simulink model "sm_car_4post_testrig"  (R2021b)
settings: Solver=ode23t  StartTime=0.0  StopTime=20  MaxStep=0.4  RelTol=1e-3  AbsTol=1e-3  EnableMultiTasking=on
PreLoadFcn:
  | sm_car_4post_param
  | sm_car_4post_param_posts
  | load sm_car_4post_op_01
  | load sm_car_4post_op_02
  | load sm_car_4post_op_03
  | 
  | 
  | sm_car_4post_vehicle_01_data
  | sm_car_4post_vehicle_02_data
  | sm_car_4post_vehicle_03_data
  | sm_car_4post_init_data
  | Vehicle = Vehicle_01;
  | sm_car_4post_op = sm_car_4post_op_01;
values from neighbouring files (symbols this model uses):
  brake_pressure_factor = 0.1    [sm_car_4post_param.m]
  brake_rear_factor = 0.3    [sm_car_4post_param.m]
  Init = struct    [sm_car_4post_init_data.m]
  N = 100    [sm_extr_data_cam_roller_curve.m]
  s = sin(q)    [sm_extr_data_cam_roller_curve.m]
  sm_car_4post_op_01 = simscape.op.create(simlog_sm_car_4post,20)    [sm_car_4post_gen_op.m]
  Vehicle_01 = struct    [sm_car_4post_vehicle_01_data.m]
undefined symbols (not defined in the file or in its folder): Axle, Hub, ShaftF, ShaftR, smcar_param, X, xy_data_car_side, xy_data_membrane, Y, Z
libraries: fl_lib x68, sm_lib x50, nesl_utility x40, sm_car_4post_lib x34, simulink x2
(part 2 of 4)

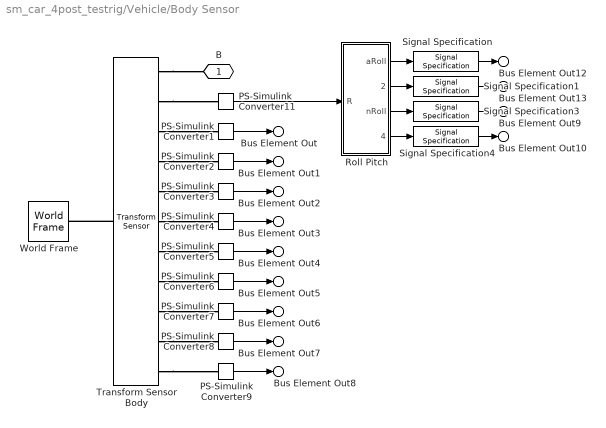
== system sm_car_4post_testrig/Vehicle/Body Sensor ==
  PS-Simulink Converter1 : nesl_utility/PS-Simulink Converter  PhysicalDomain=network_engine_domain  SubClassName=ps_output  LeftPortType=input  RightPortType=output  PseudoPeriodic=off  Frequencies=[]  Unit=m  AffineConversion=off
      settings: SourceProductBaseCode=PW,SS
  PS-Simulink Converter11 : nesl_utility/PS-Simulink Converter  PhysicalDomain=network_engine_domain  SubClassName=ps_output  LeftPortType=input  RightPortType=output  PseudoPeriodic=off  Frequencies=[]  Unit=1  AffineConversion=off
      settings: SourceProductBaseCode=PW,SS
  PS-Simulink Converter2 : nesl_utility/PS-Simulink Converter  PhysicalDomain=network_engine_domain  SubClassName=ps_output  LeftPortType=input  RightPortType=output  PseudoPeriodic=off  Frequencies=[]  Unit=m  AffineConversion=off
      settings: SourceProductBaseCode=PW,SS
  PS-Simulink Converter3 : nesl_utility/PS-Simulink Converter  PhysicalDomain=network_engine_domain  SubClassName=ps_output  LeftPortType=input  RightPortType=output  PseudoPeriodic=off  Frequencies=[]  Unit=m  AffineConversion=off
      settings: SourceProductBaseCode=PW,SS
  PS-Simulink Converter4 : nesl_utility/PS-Simulink Converter  PhysicalDomain=network_engine_domain  SubClassName=ps_output  LeftPortType=input  RightPortType=output  PseudoPeriodic=off  Frequencies=[]  Unit=m/s  AffineConversion=off
      settings: SourceProductBaseCode=PW,SS
  PS-Simulink Converter5 : nesl_utility/PS-Simulink Converter  PhysicalDomain=network_engine_domain  SubClassName=ps_output  LeftPortType=input  RightPortType=output  PseudoPeriodic=off  Frequencies=[]  Unit=m/s  AffineConversion=off
      settings: SourceProductBaseCode=PW,SS
  PS-Simulink Converter6 : nesl_utility/PS-Simulink Converter  PhysicalDomain=network_engine_domain  SubClassName=ps_output  LeftPortType=input  RightPortType=output  PseudoPeriodic=off  Frequencies=[]  Unit=m/s  AffineConversion=off
      settings: SourceProductBaseCode=PW,SS
  PS-Simulink Converter7 : nesl_utility/PS-Simulink Converter  PhysicalDomain=network_engine_domain  SubClassName=ps_output  LeftPortType=input  RightPortType=output  PseudoPeriodic=off  Frequencies=[]  Unit=m/s^2  AffineConversion=off
      settings: SourceProductBaseCode=PW,SS
  PS-Simulink Converter8 : nesl_utility/PS-Simulink Converter  PhysicalDomain=network_engine_domain  SubClassName=ps_output  LeftPortType=input  RightPortType=output  PseudoPeriodic=off  Frequencies=[]  Unit=m/s^2  AffineConversion=off
      settings: SourceProductBaseCode=PW,SS
  PS-Simulink Converter9 : nesl_utility/PS-Simulink Converter  PhysicalDomain=network_engine_domain  SubClassName=ps_output  LeftPortType=input  RightPortType=output  PseudoPeriodic=off  Frequencies=[]  Unit=m/s^2  AffineConversion=off
      settings: SourceProductBaseCode=PW,SS
  Roll Pitch : Subsystem
  Signal Specification : SignalSpecification  Unit=rad
  Signal Specification1 : SignalSpecification  Unit=rad
  Signal Specification3 : SignalSpecification  Unit=rad/s
  Signal Specification4 : SignalSpecification  Unit=rad/s
  Transform Sensor Body : sm_lib/Frames and Transforms/Transform Sensor  MeasurementFrame=NonRotatingFollower  SenseAngle=off  SenseAxis=off  SenseAngle1=off  SenseAngle2=off  SenseAngle3=off  SenseQ=off  SenseR=on  SenseOmegaX=off  SenseOmegaY=off  SenseOmegaZ=off  SenseOmega1=off  SenseOmega2=off  SenseOmega3=off  SenseQDot=off  SenseRDot=off  SenseAlphaX=off  SenseAlphaY=off  SenseAlphaZ=off  SenseAlpha1=off  SenseAlpha2=off  SenseAlpha3=off  SenseQDDot=off  SenseRDDot=off  SenseX=on  SenseY=on  SenseZ=on  SenseRad=off  SenseAzim=off  SenseDist=off  SenseInc=off  SenseXDot=on  SenseYDot=on  SenseZDot=on  SenseRadDot=off  SenseAzimDot=off  SenseDistDot=off  SenseIncDot=off  SenseXDDot=on  SenseYDDot=on  SenseZDDot=on  SenseRadDDot=off  SenseAzimDDot=off  SenseDistDDot=off  SenseIncDDot=off
  World Frame : sm_lib/Frames and Transforms/World Frame
  B : PMIOPort  Side=Left
  Bus Element Out : Outport  VectorParamsAs1DForOutWhenUnconnected=off  PortName=Body  Element=x
  Bus Element Out1 : Outport  VectorParamsAs1DForOutWhenUnconnected=off  PortName=Body  Element=y
  Bus Element Out2 : Outport  VectorParamsAs1DForOutWhenUnconnected=off  PortName=Body  Element=z
  Bus Element Out3 : Outport  VectorParamsAs1DForOutWhenUnconnected=off  PortName=Body  Element=vx
  Bus Element Out4 : Outport  VectorParamsAs1DForOutWhenUnconnected=off  PortName=Body  Element=vy
  Bus Element Out5 : Outport  VectorParamsAs1DForOutWhenUnconnected=off  PortName=Body  Element=vz
  Bus Element Out6 : Outport  VectorParamsAs1DForOutWhenUnconnected=off  PortName=Body  Element=gx
  Bus Element Out7 : Outport  VectorParamsAs1DForOutWhenUnconnected=off  PortName=Body  Element=gy
  Bus Element Out8 : Outport  VectorParamsAs1DForOutWhenUnconnected=off  PortName=Body  Element=gz
  Bus Element Out9 : Outport  VectorParamsAs1DForOutWhenUnconnected=off  PortName=Body  Element=nRoll
  Bus Element Out10 : Outport  VectorParamsAs1DForOutWhenUnconnected=off  PortName=Body  Element=nPitch
  Bus Element Out12 : Outport  VectorParamsAs1DForOutWhenUnconnected=off  PortName=Body  Element=aRoll
  Bus Element Out13 : Outport  VectorParamsAs1DForOutWhenUnconnected=off  PortName=Body  Element=aPitch
  wires:
  PS-Simulink Converter9/1 -> Bus Element Out8/1
  PS-Simulink Converter11/1 -> Roll Pitch/1(R)
  PS-Simulink Converter6/1 -> Bus Element Out5/1
  PS-Simulink Converter7/1 -> Bus Element Out6/1
  PS-Simulink Converter2/1 -> Bus Element Out1/1
  PS-Simulink Converter8/1 -> Bus Element Out7/1
  PS-Simulink Converter5/1 -> Bus Element Out4/1
  PS-Simulink Converter3/1 -> Bus Element Out2/1
  PS-Simulink Converter1/1 -> Bus Element Out/1
  PS-Simulink Converter4/1 -> Bus Element Out3/1
  Signal Specification/1 -> Bus Element Out12/1
  Signal Specification1/1 -> Bus Element Out13/1
  Signal Specification3/1 -> Bus Element Out9/1
  Signal Specification4/1 -> Bus Element Out10/1
  Roll Pitch/3(nRoll) -> Signal Specification3/1
  Roll Pitch/4(nPitch) -> Signal Specification4/1
  Roll Pitch/2(aPitch) -> Signal Specification1/1
  Roll Pitch/1(aRoll) -> Signal Specification/1
  connections:
  Transform Sensor Body/RConn5 -- PS-Simulink Converter3/LConn1
  Transform Sensor Body/RConn4 -- PS-Simulink Converter2/LConn1
  Transform Sensor Body/RConn11 -- PS-Simulink Converter9/LConn1
  Transform Sensor Body/RConn2 -- PS-Simulink Converter11/LConn1
  Transform Sensor Body/RConn7 -- PS-Simulink Converter5/LConn1
  Transform Sensor Body/RConn3 -- PS-Simulink Converter1/LConn1
  Transform Sensor Body/LConn1 -- World Frame/RConn1
  Transform Sensor Body/RConn1 -- B/RConn1
  Transform Sensor Body/RConn10 -- PS-Simulink Converter8/LConn1
  Transform Sensor Body/RConn9 -- PS-Simulink Converter7/LConn1
  Transform Sensor Body/RConn8 -- PS-Simulink Converter6/LConn1
  Transform Sensor Body/RConn6 -- PS-Simulink Converter4/LConn1

== system sm_car_4post_testrig/Vehicle/Brakes ==
  DrvBus : Inport
  CtrlBus : Inport  Port=2
  Pedal : Subsystem  Tag=PublishSubsystem  VariantControl=Pedal  mask(Pedal Controlled Brakes){brk_max_p_fa=Brakes.Front.Caliper.pMax.Value, brk_max_p_ra=Brakes.Rear.Caliper.pMax.Value, brk_filt_fa=1/Brakes.Front.Caliper.fActuatorCutoff.Value, brk_filt_ra=1/Brakes.Rear.Caliper.fActuatorCutoff.Value}
      mask help: Brakes for four-wheeled vehicle. The brake pressure varies with brake pedal travel (0-1).
      mask TypeOptions brk_max_p_fa: Actuator FL/brk_max_p | Actuator FR/brk_max_p
      mask TypeOptions brk_max_p_ra: Actuator RL/brk_max_p | Actuator RR/brk_max_p
      mask TypeOptions brk_filt_fa: Actuator FL/brk_filt | Actuator FR/brk_filt
      mask TypeOptions brk_filt_ra: Actuator RL/brk_filt | Actuator RR/brk_filt
      mask DialogControl cont_brakes Prompt: Brakes
      mask DialogControl cont_brk_act Prompt: Actuator
      mask DialogControl text_brakes_maxp Prompt: Max Pad Pressure (Pa)
      mask DialogControl text_brakes_filt Prompt: Time Constant (s)
  FL : PMIOPort  Side=Left
  FR : PMIOPort  Port=2  Side=Right
  RL : PMIOPort  Port=3  Side=Left
  RR : PMIOPort  Port=4  Side=Right
  BrakeOut : Outport  VectorParamsAs1DForOutWhenUnconnected=off
  wires:
  DrvBus/1 -> Pedal/1(DrvBus)
  Pedal/1(BrakeOut) -> BrakeOut/1
  CtrlBus/1 -> Pedal/2(CtrlBus)
  connections:
  Pedal/LConn1 -- FL/RConn1
  Pedal/RConn2 -- RR/RConn1
  Pedal/LConn2 -- RL/RConn1
  Pedal/RConn1 -- FR/RConn1

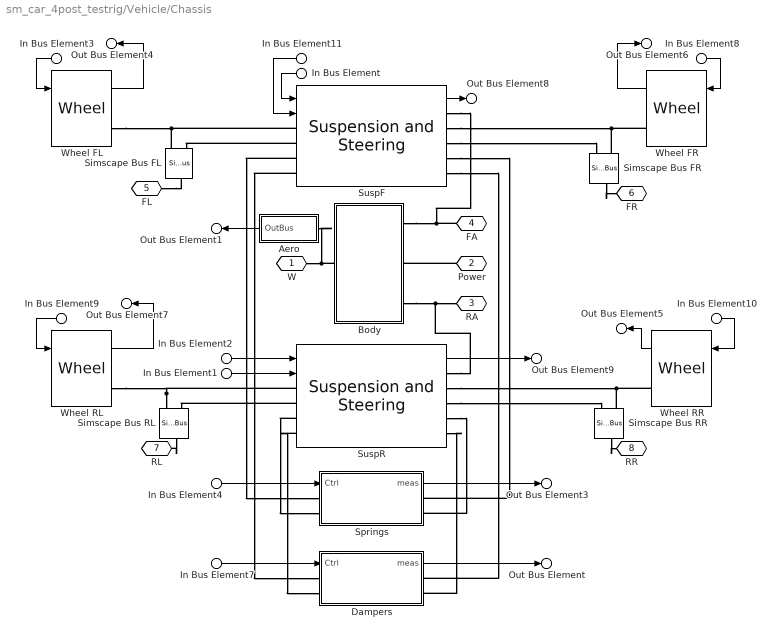
== system sm_car_4post_testrig/Vehicle/Chassis ==
  In Bus Element11 : Inport  PortName=DrvBus
  In Bus Element1 : Inport  PortName=DrvBus
  In Bus Element3 : Inport  Port=2  PortName=RdBus  Element=FL
  In Bus Element8 : Inport  Port=2  PortName=RdBus  Element=FR
  In Bus Element10 : Inport  Port=2  PortName=RdBus  Element=RR
  In Bus Element9 : Inport  Port=2  PortName=RdBus  Element=RL
  In Bus Element7 : Inport  Port=3  PortName=CtrlBus  Element=Damper
  In Bus Element : Inport  Port=3  PortName=CtrlBus  Element=SuspF
  In Bus Element2 : Inport  Port=3  PortName=CtrlBus  Element=SuspR
  In Bus Element4 : Inport  Port=3  PortName=CtrlBus  Element=Spring
  Aero : Subsystem  mask{CL=Chassis.Aero.CL.Value, CD=Chassis.Aero.CD.Value, rho=Chassis.Aero.rho_air.Value, A=Chassis.Aero.ARef.Value, sCentreOfPressure=Chassis.Aero.sPressureCentre.Value}
      mask prompts: CL "Lift Coeff (-)"; CD "Drag Coeff (-)"; rho "Air Density (kg/m^3)"; A "Reference Area (m^2)"; sCentreOfPressure "Centre of Pressure [xyz] (m)"
  Body : Subsystem  mask{hp_mount_fa=Chassis.Body.sAxleF.Value, hp_mount_ra=Chassis.Body.sAxleR.Value, hp_mount_power=Chassis.Body.sPower.Value, hp_chassis_cg=Chassis.Body.sCG.Value, chassis_mass=Chassis.Body.m.Value, chassis_inertia=Chassis.Body.J.Value, clr_chassis_hp_cg=smcar_param.hp.clr, opc_chassis_hp_cg=smcar_param.hp.opc, size_chassis_hp_cg=smcar_param.hp.rad, body_geo_hp=smcar_param.body.hp, whl_cutout_rad=0.5, whl_base=abs(Chassis.Body.sAxleF.Value(1)-Chassis.Body.sAxleR.Value(1)), thk_top=0.05, thk_side=0.05, car_track=Chassis.Body.Width.Value, extr_data_emblem_f=xy_data_membrane*0.2, extr_data_emblem_r=xy_data_membrane*0.2, clr_body_geo_top=smcar_param.blue, opc_body_geo_top=0.3*smcar_param.part.opc, clr_body_geo_left=smcar_param.blue, opc_body_geo_left=0.3*smcar_param.part.opc, clr_body_geo_right=smcar_param.blue, opc_body_geo_right=0.3*smcar_param.part.opc, clr_emblem_f=smcar_param.white, opc_emblem_f=smcar_param.part.opc, clr_emblem_r=smcar_param.white, opc_emblem_r=smcar_param.part.opc}
      mask prompts: hp_mount_power "HP Power [xyz] (m)"; hp_chassis_cg "Chassis CG [xyz] (m)"; chassis_mass "Mass (kg)"; chassis_inertia "Inertia [Ixx Iyy Izz]"; body_geo_hp "Body Geometry HP [xyz] (m)"; whl_cutout_rad "Wheel Cutout Radius (m)"; whl_base "Wheelbase (m)"; thk_top "Top Thickness (m)"; thk_side "Side Thickness (m)"; car_track "Width (m)"; extr_data_emblem_f "Emblem Data Front [xy] (m)"; extr_data_emblem_r "Emblem Data Rear [xy] (m)"
      mask TypeOptions hp_mount_fa:
      | Transform
      | Front Mount/TranslationCartesianOffset
      mask TypeOptions hp_mount_ra:
      | Transform
      | Rear Mount/TranslationCartesianOffset
      mask TypeOptions hp_mount_power:
      | Transform
      | Power Mount/TranslationCartesianOffset
      mask TypeOptions hp_chassis_cg:
      | Transform
      | Body CG/TranslationCartesianOffset
      mask TypeOptions chassis_mass:
      | Body Mass
      | and Inertia/Mass
      mask TypeOptions chassis_inertia:
      | Body Mass
      | and Inertia/MomentsOfInertia
      mask TypeOptions clr_chassis_hp_cg:
      | Body Mass
      | and Inertia/GraphicDiffuseColor | Vis HP Mount Front/GraphicDiffuseColor | Vis HP Mount Rear/GraphicDiffuseColor
      mask TypeOptions opc_chassis_hp_cg:
      | Body Mass
      | and Inertia/GraphicOpacity | Vis HP Mount Front/GraphicOpacity | Vis HP Mount Rear/GraphicOpacity
      mask TypeOptions size_chassis_hp_cg:
      | Body Mass
      | and Inertia/SphereRadius | Vis HP Mount Front/SphereRadius | Vis HP Mount Rear/SphereRadius
      mask TypeOptions body_geo_hp:
      | Transform
      | Body/TranslationCartesianOffset
      mask TypeOptions whl_cutout_rad:
      | Body
      | Geometry/whl_cutout_rad
      mask TypeOptions whl_base:
      | Body
      | Geometry/whl_base
      mask TypeOptions thk_top:
      | Body
      | Geometry/thk_top
      mask TypeOptions thk_side:
      | Body
      | Geometry/thk_side
      mask TypeOptions car_track:
      | Body
      | Geometry/car_track
      mask TypeOptions extr_data_emblem_f:
      | Body
      | Geometry/extr_data_emblem_f
      mask TypeOptions extr_data_emblem_r:
      | Body
      | Geometry/extr_data_emblem_r
      mask TypeOptions clr_body_geo_top:
      | Body
      | Geometry/clr_body_geo_top
      mask TypeOptions opc_body_geo_top:
      | Body
      | Geometry/opc_body_geo_top
      mask TypeOptions clr_body_geo_left:
      | Body
      | Geometry/clr_body_geo_left
      mask TypeOptions opc_body_geo_left:
      | Body
      | Geometry/opc_body_geo_left
      mask TypeOptions clr_body_geo_right:
      | Body
      | Geometry/clr_body_geo_right
      mask TypeOptions opc_body_geo_right:
      | Body
      | Geometry/opc_body_geo_right
      mask TypeOptions clr_emblem_f:
      | Body
      | Geometry/clr_emblem_f
      mask TypeOptions opc_emblem_f:
      | Body
      | Geometry/opc_emblem_f
      mask TypeOptions clr_emblem_r:
      | Body
      | Geometry/clr_emblem_r
      mask TypeOptions opc_emblem_r:
      | Body
      | Geometry/opc_emblem_r
      mask DialogControl cont_chassis Prompt: Chassis
      mask DialogControl text_chassis_mount_hp_blank Prompt: [xyz] (m)
      mask DialogControl text_chassis_fa Prompt: Front Susp.
      mask DialogControl text_chassis_ra Prompt: Rear Susp.
      mask DialogControl text_chassis_hp_mount Prompt: HP Mount
      mask DialogControl cont_chassis_vis Prompt: Visualization
      mask DialogControl text_chassis_vis_clr Prompt: Color [RGB]
      mask DialogControl text_chassis_vis_opc Prompt: Opacity (0-1)
      mask DialogControl text_chassis_vis_size Prompt: Size [xyz] (m)
      mask DialogControl text_chassis_vis_hp Prompt: Hardpoints
      mask DialogControl cont_body_geometry Prompt: Body
      mask DialogControl cont_body_geo_vis Prompt: Visualization
      mask DialogControl text_body_geo_clr Prompt: Color [RGB]
      mask DialogControl text_body_geo_opc Prompt: Opac. (0-1)
      mask DialogControl text_vis_body_geo_top Prompt: Top
      mask DialogControl text_vis_body_geo_l Prompt: Left Side
      mask DialogControl text_vis_body_geo_r Prompt: Right Side
      mask DialogControl text_vis_body_emblem_f Prompt: Emblem Front
      mask DialogControl text_vis_body_emblem_r Prompt: Emblem Rear
      mask Display: image(fullfile(matlabroot,'toolbox','physmod','sm','smdemos','car_4post_testrig','images','sm_car_4post_body_IMAGE.png'));
  Dampers : Subsystem  mask{Damper=Chassis.Damper}
      mask prompts: Damper "Damper Parameters"
      mask Display: image(fullfile(matlabroot,'toolbox','physmod','sm','smdemos','car_4post_testrig','images','sm_car_4post_damper_IMAGE.png'));
  Simscape Bus FL : SimscapeBus  HierarchyStrings=Axle;Hub
  Simscape Bus FR : SimscapeBus  HierarchyStrings=Hub;Axle
  Simscape Bus RL : SimscapeBus  HierarchyStrings=Axle;Hub
  Simscape Bus RR : SimscapeBus  HierarchyStrings=Hub;Axle
  Springs : Subsystem  mask{Spring=Vehicle.Chassis.Spring}
      mask prompts: Spring "Spring Parameters"
      mask Display: image(fullfile(matlabroot,'toolbox','physmod','sm','smdemos','car_4post_testrig','images','sm_car_4post_spring_IMAGE.png'));
  SuspF : sm_car_4post_lib/Suspension and Steering  Susp=Chassis.SuspF  Init=Init.Front  InitTriggerDropdown=1
      settings: SourceProductBaseCode=MS
  SuspR : sm_car_4post_lib/Suspension and Steering  Susp=Chassis.SuspR  Init=Init.Rear  InitTriggerDropdown=1
      settings: SourceProductBaseCode=MS
  Wheel FL : sm_car_4post_lib/Wheel  popup_leftRight=Left  Tire=Chassis.TyreF
      settings: SourceProductBaseCode=MS
  Wheel FR : sm_car_4post_lib/Wheel  popup_leftRight=Right  Tire=Chassis.TyreF
      settings: SourceProductBaseCode=MS
  Wheel RL : sm_car_4post_lib/Wheel  popup_leftRight=Left  Tire=Chassis.TyreR
      settings: SourceProductBaseCode=MS
  Wheel RR : sm_car_4post_lib/Wheel  popup_leftRight=Right  Tire=Chassis.TyreR
      settings: SourceProductBaseCode=MS
  W : PMIOPort  Side=Right
  Power : PMIOPort  Port=2  Side=Right
  RA : PMIOPort  Port=3  Side=Right
  FA : PMIOPort  Port=4  Side=Left
  FL : PMIOPort  Port=5  Side=Left
  FR : PMIOPort  Port=6  Side=Right
  RL : PMIOPort  Port=7  Side=Left
  RR : PMIOPort  Port=8  Side=Right
  Out Bus Element4 : Outport  VectorParamsAs1DForOutWhenUnconnected=off  PortName=VehBus  Element=WhlFL
  Out Bus Element6 : Outport  VectorParamsAs1DForOutWhenUnconnected=off  PortName=VehBus  Element=WhlFR
  Out Bus Element5 : Outport  VectorParamsAs1DForOutWhenUnconnected=off  PortName=VehBus  Element=WhlRR
  Out Bus Element7 : Outport  VectorParamsAs1DForOutWhenUnconnected=off  PortName=VehBus  Element=WhlRL
  Out Bus Element1 : Outport  VectorParamsAs1DForOutWhenUnconnected=off  PortName=VehBus  Element=Aero
  Out Bus Element : Outport  VectorParamsAs1DForOutWhenUnconnected=off  PortName=VehBus  Element=Damper
  Out Bus Element3 : Outport  VectorParamsAs1DForOutWhenUnconnected=off  PortName=VehBus  Element=Spring
  Out Bus Element8 : Outport  VectorParamsAs1DForOutWhenUnconnected=off  PortName=VehBus  Element=SuspF
  Out Bus Element9 : Outport  VectorParamsAs1DForOutWhenUnconnected=off  PortName=VehBus  Element=SuspR
  wires:
  Springs/1(meas) -> Out Bus Element3/1
  Dampers/1(meas) -> Out Bus Element/1
  In Bus Element3/1 -> Wheel FL/1
  Wheel FR/1 -> Out Bus Element6/1
  In Bus Element10/1 -> Wheel RR/1
  Wheel RL/1 -> Out Bus Element7/1
  In Bus Element8/1 -> Wheel FR/1
  Wheel FL/1 -> Out Bus Element4/1
  In Bus Element9/1 -> Wheel RL/1
  Wheel RR/1 -> Out Bus Element5/1
  In Bus Element11/1 -> SuspF/2
  SuspF/1 -> Out Bus Element8/1
  In Bus Element/1 -> SuspF/1
  In Bus Element1/1 -> SuspR/2
  SuspR/1 -> Out Bus Element9/1
  In Bus Element2/1 -> SuspR/1
  In Bus Element7/1 -> Dampers/1(Ctrl)
  In Bus Element4/1 -> Springs/1(Ctrl)
  Aero/1(OutBus) -> Out Bus Element1/1
  connections:
  Aero/LConn1 -- Body/LConn1 -- W/RConn1
  Body/RConn3 -- SuspR/RConn1 -- RA/RConn1
  Simscape Bus RR/RConn1 -- RR/RConn1
  FL/RConn1 -- Simscape Bus FL/RConn1
  Simscape Bus FR/RConn1 -- FR/RConn1
  Simscape Bus RL/RConn1 -- RL/RConn1
  Simscape Bus FR/LConn2 -- Wheel FR/RConn1 -- SuspF/RConn2
  Simscape Bus FL/LConn1 -- Wheel FL/RConn1 -- SuspF/LConn1
  FA/RConn1 -- SuspF/RConn1 -- Body/RConn1
  SuspF/LConn2 -- Simscape Bus FL/LConn2
  SuspF/RConn3 -- Simscape Bus FR/LConn1
  SuspF/LConn3 -- Springs/LConn1
  SuspF/RConn4 -- Springs/RConn1
  SuspF/LConn4 -- Dampers/LConn1
  SuspF/RConn5 -- Dampers/RConn1
  Simscape Bus RL/LConn1 -- Wheel RL/RConn1 -- SuspR/LConn1
  Simscape Bus RR/LConn2 -- Wheel RR/RConn1 -- SuspR/RConn2
  SuspR/LConn2 -- Simscape Bus RL/LConn2
  SuspR/RConn3 -- Simscape Bus RR/LConn1
  SuspR/LConn3 -- Springs/LConn2
  SuspR/RConn4 -- Springs/RConn2
  SuspR/LConn4 -- Dampers/LConn2
  SuspR/RConn5 -- Dampers/RConn2
  Power/RConn1 -- Body/RConn2

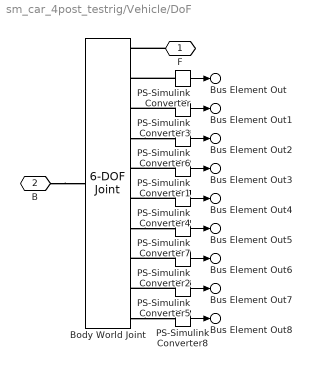
== system sm_car_4post_testrig/Vehicle/DoF ==
  Body World Joint : sm_lib/Joints/6-DOF Joint  JointMode=Normal  SenseConstraintForce=off  SenseConstraintForceX=off  SenseConstraintForceY=off  SenseConstraintForceZ=off  SenseConstraintTorque=off  SenseConstraintTorqueX=off  SenseConstraintTorqueY=off  SenseConstraintTorqueZ=off  SenseTotalForce=off  SenseTotalForceX=off  SenseTotalForceY=off  SenseTotalForceZ=off  SenseTotalTorque=off  SenseTotalTorqueX=off  SenseTotalTorqueY=off  SenseTotalTorqueZ=off  CompositeWrenchDir=FollowerOnBase  CompositeWrenchFrame=BaseFrame  PxEquilibriumPosition=0  PxEquilibriumPositionUnits=m  PxSpringStiffness=0  PxSpringStiffnessUnits=N/m  PxDampingCoefficient=0  PxDampingCoefficientUnits=N/(m/s)  PxTorqueActuationMode=NoTorque  PxMotionActuationMode=ComputedMotion  PxSensePosition=on  PxSenseVelocity=on  PxSenseAcceleration=on  PxSenseTorqueForce=off  PxSenseLowerLimitTorqueForce=off  PxSenseUpperLimitTorqueForce=off  PxLowerLimitSpecify=off  PxLowerLimitBound=-1  PxLowerLimitBoundUnits=m  PxLowerLimitStiffness=1e6  PxLowerLimitStiffnessUnits=N/m  PxLowerLimitDamping=1e3  PxLowerLimitDampingUnits=N/(m/s)  PxLowerLimitTransitionRegionWidth=1e-4  PxLowerLimitTransitionRegionWidthUnits=m  PxUpperLimitSpecify=off  PxUpperLimitBound=1  PxUpperLimitBoundUnits=m  PxUpperLimitStiffness=1e6  PxUpperLimitStiffnessUnits=N/m  PxUpperLimitDamping=1e3  PxUpperLimitDampingUnits=N/(m/s)  PxUpperLimitTransitionRegionWidth=1e-4  PxUpperLimitTransitionRegionWidthUnits=m  PxPositionTargetSpecify=on  PxPositionTargetPriority=Low  PxPositionTargetValue=Init.sChassis.Value(1)  PxPositionTargetValueUnits=m  PxVelocityTargetSpecify=on  PxVelocityTargetPriority=Low  PxVelocityTargetValue=Init.vChassis.Value(1)  PxVelocityTargetValueUnits=m/s  PyEquilibriumPosition=0  PyEquilibriumPositionUnits=m  PySpringStiffness=0  PySpringStiffnessUnits=N/m  PyDampingCoefficient=0  PyDampingCoefficientUnits=N/(m/s)  PyTorqueActuationMode=NoTorque  PyMotionActuationMode=ComputedMotion  PySensePosition=on  PySenseVelocity=on  PySenseAcceleration=on  PySenseTorqueForce=off  PySenseLowerLimitTorqueForce=off  PySenseUpperLimitTorqueForce=off  PyLowerLimitSpecify=off  PyLowerLimitBound=-1  PyLowerLimitBoundUnits=m  PyLowerLimitStiffness=1e6  PyLowerLimitStiffnessUnits=N/m  PyLowerLimitDamping=1e3  PyLowerLimitDampingUnits=N/(m/s)  PyLowerLimitTransitionRegionWidth=1e-4  PyLowerLimitTransitionRegionWidthUnits=m  PyUpperLimitSpecify=off  PyUpperLimitBound=1  PyUpperLimitBoundUnits=m  PyUpperLimitStiffness=1e6  PyUpperLimitStiffnessUnits=N/m  PyUpperLimitDamping=1e3  PyUpperLimitDampingUnits=N/(m/s)  PyUpperLimitTransitionRegionWidth=1e-4  PyUpperLimitTransitionRegionWidthUnits=m  PyPositionTargetSpecify=on  PyPositionTargetPriority=Low  PyPositionTargetValue=Init.sChassis.Value(2)  PyPositionTargetValueUnits=m  PyVelocityTargetSpecify=on  PyVelocityTargetPriority=Low  PyVelocityTargetValue=Init.vChassis.Value(2)  PyVelocityTargetValueUnits=m/s  PzEquilibriumPosition=0  PzEquilibriumPositionUnits=m  PzSpringStiffness=0  PzSpringStiffnessUnits=N/m  PzDampingCoefficient=0  PzDampingCoefficientUnits=N/(m/s)  PzTorqueActuationMode=NoTorque  PzMotionActuationMode=ComputedMotion  PzSensePosition=on  PzSenseVelocity=on  PzSenseAcceleration=on  PzSenseTorqueForce=off  PzSenseLowerLimitTorqueForce=off  PzSenseUpperLimitTorqueForce=off  PzLowerLimitSpecify=off  PzLowerLimitBound=-1  PzLowerLimitBoundUnits=m  PzLowerLimitStiffness=1e6  PzLowerLimitStiffnessUnits=N/m  PzLowerLimitDamping=1e3  PzLowerLimitDampingUnits=N/(m/s)  PzLowerLimitTransitionRegionWidth=1e-4  PzLowerLimitTransitionRegionWidthUnits=m  PzUpperLimitSpecify=off  PzUpperLimitBound=1  PzUpperLimitBoundUnits=m  PzUpperLimitStiffness=1e6  PzUpperLimitStiffnessUnits=N/m  PzUpperLimitDamping=1e3  PzUpperLimitDampingUnits=N/(m/s)  PzUpperLimitTransitionRegionWidth=1e-4  PzUpperLimitTransitionRegionWidthUnits=m  PzPositionTargetSpecify=on  PzPositionTargetPriority=Low  PzPositionTargetValue=Init.sChassis.Value(3)  PzPositionTargetValueUnits=m  PzVelocityTargetSpecify=on  PzVelocityTargetPriority=Low  PzVelocityTargetValue=Init.vChassis.Value(3)  PzVelocityTargetValueUnits=m/s  SphDefPosRotationMethod=None  SphDefPosRotationAngleUnits=deg  SphDefPosRotationStandardAxis=+Z  SphDefPosRotationAngle=0.0  SphDefPosRotationArbitraryAxis=[0 0 1]  SphDefPosFollAlignAxisA=+X  SphDefPosBaseAlignAxisA=+Y  SphDefPosFollAlignAxisB=+Y  SphDefPosBaseAlignAxisB=+Z  SphDefPosRotationSequenceAxes=FollowerAxes  SphDefPosRotationSequence=XYX  SphDefPosRotationSequenceAngles=[0 0 0]  SphDefPosRotationSequenceAnglesUnits=deg  SphDefPosRotationMatrix=[1 0 0; 0 1 0; 0 0 1]  SphEqPosRotationMethod=None  SphEqPosRotationAngleUnits=deg  SphEqPosRotationStandardAxis=+Z  SphEqPosRotationAngle=0.0  SphEqPosRotationArbitraryAxis=[0 0 1]  SphEqPosFollAlignAxisA=+X  SphEqPosBaseAlignAxisA=+Y  SphEqPosFollAlignAxisB=+Y  SphEqPosBaseAlignAxisB=+Z  SphEqPosRotationSequenceAxes=FollowerAxes  SphEqPosRotationSequence=XYX  SphEqPosRotationSequenceAngles=[0 0 0]  SphEqPosRotationSequenceAnglesUnits=deg  SphEqPosRotationMatrix=[1 0 0; 0 1 0; 0 0 1]  SphSpringStiffness=0  SphSpringStiffnessUnits=N*m/deg  SphDampingCoefficient=0  SphDampingCoefficientUnits=N*m/(deg/s)  SphActuateTorqueX=off  SphActuateTorqueY=off  SphActuateTorqueZ=off  SphActuateTorque=off  SphTorqueActuationMode=NoTorque  SphMotionActuationMode=ComputedMotion  SphActuationFrame=BaseFrame  SphSensePosition=off  SphSenseVelocityX=off  SphSenseVelocityY=off  SphSenseVelocityZ=off  SphSenseVelocity=off  SphSenseAccelerationX=off  SphSenseAccelerationY=off  SphSenseAccelerationZ=off  SphSenseAcceleration=off  SphSenseTorqueX=off  SphSenseTorqueY=off  SphSenseTorqueZ=off  SphSenseTorqueForce=off  SphSenseLowerLimitTorqueMag=off  SphSenseUpperLimitTorqueMag=off  SphSensingFrame=BaseFrame  SphLowerLimitSpecify=off  SphLowerLimitBound=15  SphLowerLimitBoundUnits=deg  SphLowerLimitStiffness=1e4  SphLowerLimitStiffnessUnits=N*m/deg  SphLowerLimitDamping=10  SphLowerLimitDampingUnits=N*m/(deg/s)  SphLowerLimitTransitionRegionWidth=0.1  SphLowerLimitTransitionRegionWidthUnits=deg  SphUpperLimitSpecify=off  SphUpperLimitBound=45  SphUpperLimitBoundUnits=deg  SphUpperLimitStiffness=1e4  SphUpperLimitStiffnessUnits=N*m/deg  SphUpperLimitDamping=10  SphUpperLimitDampingUnits=N*m/(deg/s)  SphUpperLimitTransitionRegionWidth=0.1  SphUpperLimitTransitionRegionWidthUnits=deg  SphPositionTargetRotationMethod=RotationSequence  SphPositionTargetRotationAngleUnits=deg  SphPositionTargetRotationStandardAxis=+Z  SphPositionTargetRotationAngle=0.0  SphPositionTargetRotationArbitraryAxis=[0 0 1]  SphPositionTargetFollAlignAxisA=+X  SphPositionTargetBaseAlignAxisA=+Y  SphPositionTargetFollAlignAxisB=+Y  SphPositionTargetBaseAlignAxisB=+Z  SphPositionTargetRotationSequenceAxes=BaseAxes  SphPositionTargetRotationSequence=XYZ  SphPositionTargetRotationSequenceAngles=Init.aChassis.Value  SphPositionTargetRotationSequenceAnglesUnits=deg  SphPositionTargetRotationMatrix=[1 0 0; 0 1 0; 0 0 1]  SphPositionTargetSpecify=on  SphPositionTargetPriority=Low  SphVelocityTargetValue=[0 0 0]  SphVelocityTargetValueUnits=deg/s  SphVelocityTargetSpecify=off  SphVelocityTargetPriority=High  SphVelocityTargetInFollowerFrame=on
  PS-Simulink Converter : nesl_utility/PS-Simulink Converter  PhysicalDomain=network_engine_domain  SubClassName=ps_output  LeftPortType=input  RightPortType=output  PseudoPeriodic=off  Frequencies=[]  Unit=m  AffineConversion=off
      settings: SourceProductBaseCode=PW,SS
  PS-Simulink Converter1 : nesl_utility/PS-Simulink Converter  PhysicalDomain=network_engine_domain  SubClassName=ps_output  LeftPortType=input  RightPortType=output  PseudoPeriodic=off  Frequencies=[]  Unit=m  AffineConversion=off
      settings: SourceProductBaseCode=PW,SS
  PS-Simulink Converter2 : nesl_utility/PS-Simulink Converter  PhysicalDomain=network_engine_domain  SubClassName=ps_output  LeftPortType=input  RightPortType=output  PseudoPeriodic=off  Frequencies=[]  Unit=m  AffineConversion=off
      settings: SourceProductBaseCode=PW,SS
  PS-Simulink Converter3 : nesl_utility/PS-Simulink Converter  PhysicalDomain=network_engine_domain  SubClassName=ps_output  LeftPortType=input  RightPortType=output  PseudoPeriodic=off  Frequencies=[]  Unit=m/s  AffineConversion=off
      settings: SourceProductBaseCode=PW,SS
  PS-Simulink Converter4 : nesl_utility/PS-Simulink Converter  PhysicalDomain=network_engine_domain  SubClassName=ps_output  LeftPortType=input  RightPortType=output  PseudoPeriodic=off  Frequencies=[]  Unit=m/s  AffineConversion=off
      settings: SourceProductBaseCode=PW,SS
  PS-Simulink Converter5 : nesl_utility/PS-Simulink Converter  PhysicalDomain=network_engine_domain  SubClassName=ps_output  LeftPortType=input  RightPortType=output  PseudoPeriodic=off  Frequencies=[]  Unit=m/s  AffineConversion=off
      settings: SourceProductBaseCode=PW,SS
  PS-Simulink Converter6 : nesl_utility/PS-Simulink Converter  PhysicalDomain=network_engine_domain  SubClassName=ps_output  LeftPortType=input  RightPortType=output  PseudoPeriodic=off  Frequencies=[]  Unit=m/s^2  AffineConversion=off
      settings: SourceProductBaseCode=PW,SS
  PS-Simulink Converter7 : nesl_utility/PS-Simulink Converter  PhysicalDomain=network_engine_domain  SubClassName=ps_output  LeftPortType=input  RightPortType=output  PseudoPeriodic=off  Frequencies=[]  Unit=m/s^2  AffineConversion=off
      settings: SourceProductBaseCode=PW,SS
  PS-Simulink Converter8 : nesl_utility/PS-Simulink Converter  PhysicalDomain=network_engine_domain  SubClassName=ps_output  LeftPortType=input  RightPortType=output  PseudoPeriodic=off  Frequencies=[]  Unit=m/s^2  AffineConversion=off
      settings: SourceProductBaseCode=PW,SS
  F : PMIOPort  Side=Left
  B : PMIOPort  Port=2  Side=Right
  Bus Element Out : Outport  VectorParamsAs1DForOutWhenUnconnected=off  PortName=World  Element=x
  Bus Element Out3 : Outport  VectorParamsAs1DForOutWhenUnconnected=off  PortName=World  Element=y
  Bus Element Out6 : Outport  VectorParamsAs1DForOutWhenUnconnected=off  PortName=World  Element=z
  Bus Element Out1 : Outport  VectorParamsAs1DForOutWhenUnconnected=off  PortName=World  Element=vx
  Bus Element Out4 : Outport  VectorParamsAs1DForOutWhenUnconnected=off  PortName=World  Element=vy
  Bus Element Out7 : Outport  VectorParamsAs1DForOutWhenUnconnected=off  PortName=World  Element=vz
  Bus Element Out2 : Outport  VectorParamsAs1DForOutWhenUnconnected=off  PortName=World  Element=gx
  Bus Element Out5 : Outport  VectorParamsAs1DForOutWhenUnconnected=off  PortName=World  Element=gy
  Bus Element Out8 : Outport  VectorParamsAs1DForOutWhenUnconnected=off  PortName=World  Element=gz
  wires:
  PS-Simulink Converter1/1 -> Bus Element Out3/1
  PS-Simulink Converter/1 -> Bus Element Out/1
  PS-Simulink Converter2/1 -> Bus Element Out6/1
  PS-Simulink Converter6/1 -> Bus Element Out2/1
  PS-Simulink Converter3/1 -> Bus Element Out1/1
  PS-Simulink Converter4/1 -> Bus Element Out4/1
  PS-Simulink Converter5/1 -> Bus Element Out7/1
  PS-Simulink Converter7/1 -> Bus Element Out5/1
  PS-Simulink Converter8/1 -> Bus Element Out8/1
  connections:
  PS-Simulink Converter2/LConn1 -- Body World Joint/RConn8
  F/RConn1 -- Body World Joint/RConn1
  Body World Joint/RConn10 -- PS-Simulink Converter8/LConn1
  Body World Joint/RConn4 -- PS-Simulink Converter6/LConn1
  B/RConn1 -- Body World Joint/LConn1
  PS-Simulink Converter/LConn1 -- Body World Joint/RConn2
  PS-Simulink Converter3/LConn1 -- Body World Joint/RConn3
  PS-Simulink Converter4/LConn1 -- Body World Joint/RConn6
  PS-Simulink Converter1/LConn1 -- Body World Joint/RConn5
  Body World Joint/RConn7 -- PS-Simulink Converter7/LConn1
  PS-Simulink Converter5/LConn1 -- Body World Joint/RConn9

== system sm_car_4post_testrig/Vehicle/Powertrain ==
  CtrlD : Inport
  CtrlP : Inport  Port=2
  Driveline : Subsystem  Tag=PublishSubsystem  VariantControl=Shaft  mask(Driveline){Driveline=Powertrain.Driveline, InitTriggerDropdown=1}
      mask prompts: Driveline "Driveline Parameters"; InitTriggerDropdown "Initialization Trigger Dropdown"
      mask help: Driveline model for vehicle.
      mask init:
      | curblk = gcb;
      | 
      | % Trigger Mask Initialization for 
      | % variant subsystems below this level
      | sm_car_4post_lib_maskInitTrigger(curblk)
      mask TypeOptions InitTriggerDropdown: 0 | 1
  Power : Subsystem  mask(Power Source with Shaft Output){Power=Powertrain.Power}
      mask prompts: Power "Power Parameters"
      mask help: Power source for vehicle.
  FA : PMIOPort  Side=Left
  RA : PMIOPort  Port=2  Side=Right
  FR : PMIOPort  Port=3  Side=Right
  FL : PMIOPort  Port=4  Side=Left
  RL : PMIOPort  Port=5  Side=Left
  RR : PMIOPort  Port=6  Side=Right
  o : PMIOPort  Port=7  Side=Left
  Ref : PMIOPort  Port=8  Side=Right
  OutD : Outport  VectorParamsAs1DForOutWhenUnconnected=off
  OutP : Outport  Port=2  VectorParamsAs1DForOutWhenUnconnected=off
  wires:
  CtrlP/1 -> Power/1(CtrlBus)
  Power/1(PowerOut) -> OutP/1
  CtrlD/1 -> Driveline/1(CtrlBus)
  Driveline/1(DriveOut) -> OutD/1
  connections:
  Driveline/RConn4 -- o/RConn1
  Driveline/LConn3 -- RL/RConn1
  Driveline/RConn3 -- RR/RConn1
  Driveline/RConn2 -- FR/RConn1
  Driveline/LConn2 -- FL/RConn1
  Power/LConn1 -- Driveline/LConn4
  Driveline/RConn1 -- RA/RConn1
  Power/RConn1 -- Ref/RConn1
  Driveline/LConn1 -- FA/RConn1

== system sm_car_4post_testrig/Control/Susp/Steer ==
  Bus Creator : BusCreator  Inputs=1
  Constant : Constant  Value=0
  Steer : Outport  VectorParamsAs1DForOutWhenUnconnected=off
  wires:
  Bus Creator/1 -> Steer/1  "Steer"
  Constant/1 -> Bus Creator/1  "iMotor"

== system sm_car_4post_testrig/Vehicle/Body Sensor/Roll Pitch ==
  R : Inport
  Calculate aPitch : Subsystem
  Calculate aRoll : Subsystem
  "Flip sign for -x axis " : Gain  Gain=-1
  Select x axis : Selector  NumberOfDimensions=2  InputPortWidth=2  IndexOptions=Index vector (dialog),Index vector (dialog)  Indices=[1 2 3],1  OutputSizes=1,1
  Select y axis : Selector  NumberOfDimensions=2  InputPortWidth=2  IndexOptions=Index vector (dialog),Index vector (dialog)  Indices=[1 2 3],2  OutputSizes=1,1
  Transfer Fcn : TransferFcn  Numerator=[1 0]  Denominator=[0.01 1]
  Transfer Fcn1 : TransferFcn  Numerator=[1 0]  Denominator=[0.01 1]
  aRoll : Outport  VectorParamsAs1DForOutWhenUnconnected=off
  aPitch : Outport  Port=2  VectorParamsAs1DForOutWhenUnconnected=off
  nRoll : Outport  Port=3  VectorParamsAs1DForOutWhenUnconnected=off
  nPitch : Outport  Port=4  VectorParamsAs1DForOutWhenUnconnected=off
  wires:
  Calculate aPitch/1(Angle) -> "Flip sign for -x axis "/1
  Select x axis/1 -> Calculate aPitch/2(uvec)
  R/1 -> Select y axis/1, Select x axis/1
  Select y axis/1 -> Calculate aRoll/1(uvec)
  "Flip sign for -x axis "/1 -> Transfer Fcn1/1, aPitch/1
  Calculate aRoll/1(Angle) -> Transfer Fcn/1, aRoll/1, Calculate aPitch/1(Roll Angle)
  Transfer Fcn/1 -> nRoll/1
  Transfer Fcn1/1 -> nPitch/1

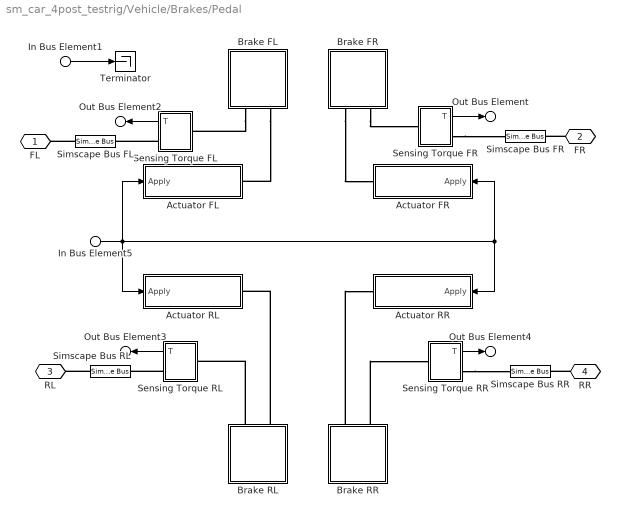
== system sm_car_4post_testrig/Vehicle/Brakes/Pedal ==
  In Bus Element5 : Inport  PortName=DrvBus  Element=rBrakePedal
  In Bus Element1 : Inport  Port=2  PortName=CtrlBus
  Actuator FL : Subsystem  mask{brk_max_p=brk_max_p_fa, brk_filt=brk_filt_fa}
      mask prompts: brk_max_p "Max Pad Pressure (Pa)"; brk_filt "Time Constant (s)"
      mask TypeOptions brk_max_p: Filter/Numerator
  Actuator FR : Subsystem  mask{brk_max_p=brk_max_p_fa, brk_filt=brk_filt_fa}
      mask prompts: brk_max_p "Max Pad Pressure (Pa)"; brk_filt "Time Constant (s)"
      mask TypeOptions brk_max_p: Filter/Numerator
  Actuator RL : Subsystem  mask{brk_max_p=brk_max_p_ra, brk_filt=brk_filt_ra}
      mask prompts: brk_max_p "Max Pad Pressure (Pa)"; brk_filt "Time Constant (s)"
      mask TypeOptions brk_max_p: Filter/Numerator
  Actuator RR : Subsystem  mask{brk_max_p=brk_max_p_ra, brk_filt=brk_filt_ra}
      mask prompts: brk_max_p "Max Pad Pressure (Pa)"; brk_filt "Time Constant (s)"
      mask TypeOptions brk_max_p: Filter/Numerator
  Brake FL : Subsystem
  Brake FR : Subsystem
  Brake RL : Subsystem
  Brake RR : Subsystem
  Sensing Torque FL : Subsystem
  Sensing Torque FR : Subsystem
  Sensing Torque RL : Subsystem
  Sensing Torque RR : Subsystem
  Simscape Bus FL : SimscapeBus  HierarchyStrings=Hub
  Simscape Bus FR : SimscapeBus  HierarchyStrings=Hub
  Simscape Bus RL : SimscapeBus  HierarchyStrings=Hub
  Simscape Bus RR : SimscapeBus  HierarchyStrings=Hub
  Terminator : Terminator
  FL : PMIOPort  Side=Left
  FR : PMIOPort  Port=2  Side=Right
  RL : PMIOPort  Port=3  Side=Left
  RR : PMIOPort  Port=4  Side=Right
  Out Bus Element2 : Outport  VectorParamsAs1DForOutWhenUnconnected=off  PortName=BrakeOut  Element=MBrakeFL
  Out Bus Element : Outport  VectorParamsAs1DForOutWhenUnconnected=off  PortName=BrakeOut  Element=MBrakeFR
  Out Bus Element3 : Outport  VectorParamsAs1DForOutWhenUnconnected=off  PortName=BrakeOut  Element=MBrakeRL
  Out Bus Element4 : Outport  VectorParamsAs1DForOutWhenUnconnected=off  PortName=BrakeOut  Element=MBrakeRR
  wires:
  In Bus Element5/1 -> Actuator RL/1(Apply), Actuator FL/1(Apply), Actuator FR/1(Apply), Actuator RR/1(Apply)
  In Bus Element1/1 -> Terminator/1
  Sensing Torque FL/1(T) -> Out Bus Element2/1
  Sensing Torque FR/1(T) -> Out Bus Element/1
  Sensing Torque RL/1(T) -> Out Bus Element3/1
  Sensing Torque RR/1(T) -> Out Bus Element4/1
  connections:
  Brake RR/LConn2 -- Sensing Torque RR/LConn1
  Brake FR/LConn2 -- Sensing Torque FR/LConn1
  Brake FR/LConn1 -- Actuator FR/RConn1
  Brake RL/LConn2 -- Actuator RL/RConn1
  Brake FL/LConn2 -- Actuator FL/RConn1
  Brake RR/LConn1 -- Actuator RR/RConn1
  FR/RConn1 -- Simscape Bus FR/RConn1
  RR/RConn1 -- Simscape Bus RR/RConn1
  Simscape Bus RL/RConn1 -- RL/RConn1
  Brake RL/LConn1 -- Sensing Torque RL/LConn1
  Simscape Bus FL/RConn1 -- FL/RConn1
  Brake FL/LConn1 -- Sensing Torque FL/LConn1
  Sensing Torque FL/RConn1 -- Simscape Bus FL/LConn1
  Sensing Torque FR/RConn1 -- Simscape Bus FR/LConn1
  Sensing Torque RL/RConn1 -- Simscape Bus RL/LConn1
  Sensing Torque RR/RConn1 -- Simscape Bus RR/LConn1

== system sm_car_4post_testrig/Vehicle/Chassis/Aero ==
  Drag : fl_lib/Physical Signals/Functions/PS Gain  gain=-0.5 * rho * CD * A N/(m^2/s^2)
  External Force and Torque : sm_lib/Forces and Torques/External Force and Torque  ForceResolutionFrame=AttachedFrame  EnableForceX=on  EnableForceY=off  EnableForceZ=on  EnableForce=off  TorqueResolutionFrame=AttachedFrame  EnableTorqueX=off  EnableTorqueY=off  EnableTorqueZ=off  EnableTorque=off
  Lift : fl_lib/Physical Signals/Functions/PS Gain  gain=-0.5 * rho * CL * A N/(m^2/s^2)
  PS Product1 : fl_lib/Physical Signals/Functions/PS Product
  PS-Simulink Converter : nesl_utility/PS-Simulink Converter  PhysicalDomain=network_engine_domain  SubClassName=ps_output  LeftPortType=input  RightPortType=output  PseudoPeriodic=off  Frequencies=[]  Unit=N  AffineConversion=off
      settings: SourceProductBaseCode=PW,SS
  PS-Simulink Converter1 : nesl_utility/PS-Simulink Converter  PhysicalDomain=network_engine_domain  SubClassName=ps_output  LeftPortType=input  RightPortType=output  PseudoPeriodic=off  Frequencies=[]  Unit=N  AffineConversion=off
      settings: SourceProductBaseCode=PW,SS
  Transform Center of Pressure : sm_lib/Frames and Transforms/Rigid Transform  TranslationMethod=Cartesian  TranslationStandardOffset=0  TranslationLengthUnit=m  TranslationStandardAxis=+Z  TranslationCartesianOffset=sCentreOfPressure  TranslationROffset=0  TranslationROffsetUnits=m  TranslationZOffset=0  TranslationZOffsetUnits=m  TranslationThetaOffset=0  TranslationThetaOffsetUnits=deg  RotationMethod=None  RotationAngleUnits=deg  RotationStandardAxis=+Z  RotationAngle=0.0  RotationArbitraryAxis=[0 0 1]  FollAlignAxisA=+X  BaseAlignAxisA=+Y  FollAlignAxisB=+Y  BaseAlignAxisB=+Z  RotationSequenceAxes=FollowerAxes  RotationSequence=XYX  RotationSequenceAngles=[0 0 0]  RotationSequenceAnglesUnits=deg  RotationMatrix=[1 0 0; 0 1 0; 0 0 1]
  Transform Sensor : sm_lib/Frames and Transforms/Transform Sensor  MeasurementFrame=Follower  SenseAngle=off  SenseAxis=off  SenseAngle1=off  SenseAngle2=off  SenseAngle3=off  SenseQ=off  SenseR=off  SenseOmegaX=off  SenseOmegaY=off  SenseOmegaZ=off  SenseOmega1=off  SenseOmega2=off  SenseOmega3=off  SenseQDot=off  SenseRDot=off  SenseAlphaX=off  SenseAlphaY=off  SenseAlphaZ=off  SenseAlpha1=off  SenseAlpha2=off  SenseAlpha3=off  SenseQDDot=off  SenseRDDot=off  SenseX=off  SenseY=off  SenseZ=off  SenseRad=off  SenseAzim=off  SenseDist=off  SenseInc=off  SenseXDot=on  SenseYDot=off  SenseZDot=off  SenseRadDot=off  SenseAzimDot=off  SenseDistDot=off  SenseIncDot=off  SenseXDDot=off  SenseYDDot=off  SenseZDDot=off  SenseRadDDot=off  SenseAzimDDot=off  SenseDistDDot=off  SenseIncDDot=off
  World Frame : sm_lib/Frames and Transforms/World Frame
  A : PMIOPort  Side=Left
  Bus Element Out1 : Outport  VectorParamsAs1DForOutWhenUnconnected=off  PortName=OutBus  Element=Fx
  Bus Element Out : Outport  VectorParamsAs1DForOutWhenUnconnected=off  PortName=OutBus  Element=Fz
  wires:
  PS-Simulink Converter1/1 -> Bus Element Out1/1
  PS-Simulink Converter/1 -> Bus Element Out/1
  connections:
  Transform Sensor/LConn1 -- World Frame/RConn1
  PS-Simulink Converter1/LConn1 -- Drag/RConn1 -- External Force and Torque/LConn1
  External Force and Torque/LConn2 -- Lift/RConn1 -- PS-Simulink Converter/LConn1
  Drag/LConn1 -- PS Product1/RConn1 -- Lift/LConn1
  Transform Sensor/RConn2 -- PS Product1/LConn1 -- PS Product1/LConn2
  Transform Center of Pressure/LConn1 -- A/RConn1
  External Force and Torque/RConn1 -- Transform Center of Pressure/RConn1 -- Transform Sensor/RConn1
